simulink model "controller_lab4"  (R2024a)
settings: Solver=FixedStepAuto  StartTime=0.0  StopTime=120  FixedStep=1/100  RelTol=1e-3  EnableMultiTasking=on
settings Model: PacingRate=10  ExtModeTrigDuration=2  Creator=DAUIN-Win10  LastModifiedBy=Alizein Khalifeh
settings OptimizationCC: EnhancedBackFolding=on  PassReuseOutputArgsAs=Individual arguments  ZeroExternalMemoryAtStartup=off  ZeroInternalMemoryAtStartup=off  MaxStackSize=64  OptimizeBlockOrder=speed  DifferentSizesBufferReuse=on  OptimizationCustomize=off  EfficientTunableParamExpr=on
settings DebuggingCC: ParameterOverflowMsg=none  ParameterTunabilityLossMsg=error  UnconnectedInputMsg=warning  UnconnectedOutputMsg=warning  UnconnectedLineMsg=warning
settings HardwareCC: ProdBitPerInt=16  ProdBitPerPointer=16  ProdBitPerSizeT=16  ProdBitPerPtrDiffT=16  ProdLargestAtomicFloat=None  ProdWordSize=8  ProdHWDeviceType=Atmel->AVR
settings ModelReferenceCC: EnableRefExpFcnMdlSchedulingChecks=on
settings SFSimCC: MATLABDynamicMemAlloc=off
settings RTWCC: Description=Embedded Coder  SystemTargetFile=ert.tlc  HardwareBoard=Arduino Uno  TemplateMakefile=ert_default_tmf  Toolchain=Arduino AVR  BuildConfiguration=Faster Runs  GPUComputeCapability=3.5  DLArmComputeVersion=19.05
settings CodeAppCC: ForceParamTrailComments=on  IgnoreCustomStorageClasses=off  OperatorAnnotations=on  SimulinkDataObjDesc=on  SFDataObjDesc=on  InsertBlockDesc=on
settings ERTTargetCC: SupportContinuousTime=on  SupportVariableSizeSignals=on  ExtModeTransport=3  ExtModeStaticAlloc=on  ExtModeAutomaticAllocSize=off  ExtModeStaticAllocSize=250  ExtModeMexFile=ext_xcp  ExtModeIntrfLevel=Level2 - Open

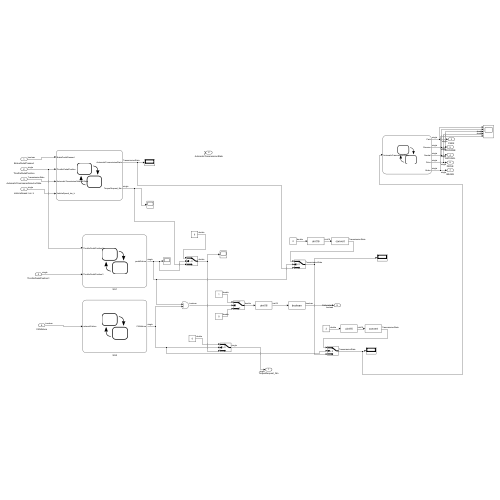
[thumbnail: Simulink's stored preview of the top-level diagram]
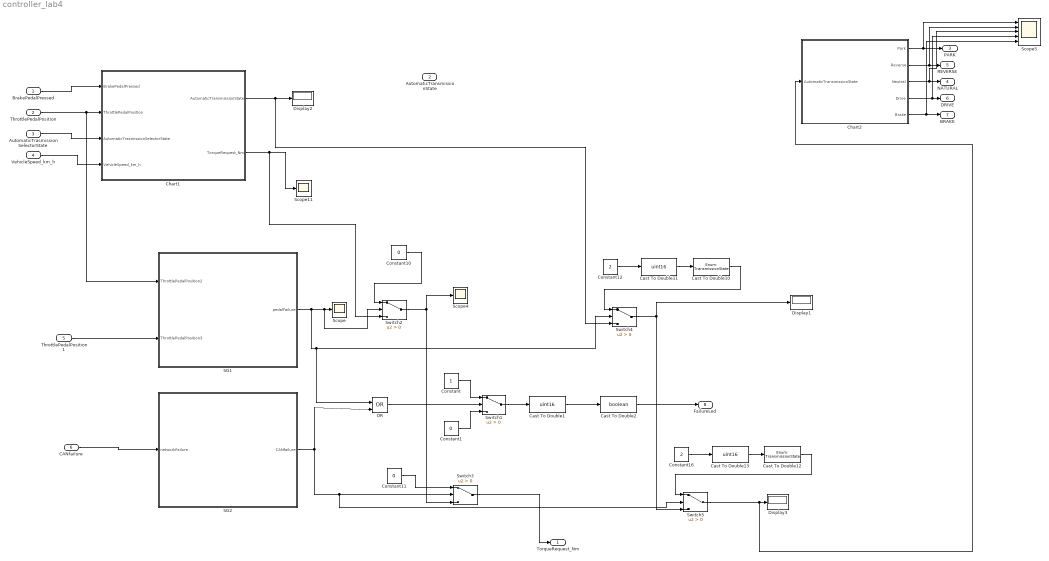
== system controller_lab4 ==
  BrakePedalPressed : Inport  OutDataTypeStr=boolean
  ThrottlePedalPosition : Inport  Port=2  OutDataTypeStr=single
  AutomaticTrasmissionSelectorState : Inport  Port=3  OutDataTypeStr=Enum: TransmissionState
  VehicleSpeed_km_h : Inport  Port=4  OutDataTypeStr=single  Unit=km/h
  ThrottlePedalPosition1 : Inport  Port=5  OutDataTypeStr=single
  CANfailure : Inport  Port=6  OutDataTypeStr=boolean
  Cast To Double1 : DataTypeConversion  OutDataTypeStr=uint16  SaturateOnIntegerOverflow=off  RndMeth=Floor
  Cast To Double10 : DataTypeConversion  OutDataTypeStr=Enum: TransmissionState  SaturateOnIntegerOverflow=off  RndMeth=Floor
  Cast To Double11 : DataTypeConversion  OutDataTypeStr=uint16  SaturateOnIntegerOverflow=off  RndMeth=Floor
  Cast To Double12 : DataTypeConversion  OutDataTypeStr=Enum: TransmissionState  SaturateOnIntegerOverflow=off  RndMeth=Floor
  Cast To Double13 : DataTypeConversion  OutDataTypeStr=uint16  SaturateOnIntegerOverflow=off  RndMeth=Floor
  Cast To Double2 : DataTypeConversion  OutDataTypeStr=boolean  SaturateOnIntegerOverflow=off  RndMeth=Floor
  Chart1 : Stateflow chart  TreatAsAtomicUnit=on
  Chart2 : Stateflow chart  TreatAsAtomicUnit=on
  Constant : Constant
  Constant1 : Constant  Value=0
  Constant10 : Constant  Value=0
  Constant11 : Constant  Value=0
  Constant12 : Constant  Value=2
  Constant16 : Constant  Value=2
  Display1 : Display
  Display2 : Display
  Display3 : Display
  OR : Logic  Operator=OR  IconShape=distinctive  AllPortsSameDT=off  OutDataTypeStr=boolean
  SG1 : Stateflow chart  TreatAsAtomicUnit=on
  SG2 : Stateflow chart  TreatAsAtomicUnit=on
  Scope : Scope
  Scope11 : Scope
  Scope4 : Scope
  Scope5 : Scope  NumInputPorts=5
  Switch{1..5} (5 alike) : Switch  Criteria=u2 > Threshold  SaturateOnIntegerOverflow=off  InputSameDT=off
  TorqueRequest_Nm : Outport  OutDataTypeStr=single  Unit=N*m
  AutomaticTransmissionState : Outport  Port=2
  PARK : Outport  Port=3  OutDataTypeStr=single  Unit=N*m
  NATURAL : Outport  Port=4  OutDataTypeStr=single  Unit=N*m
  REVERSE : Outport  Port=5  OutDataTypeStr=single  Unit=N*m
  DRIVE : Outport  Port=6  OutDataTypeStr=single  Unit=N*m
  BRAKE : Outport  Port=7  OutDataTypeStr=single  Unit=N*m
  FailureLed : Outport  Port=8  OutDataTypeStr=boolean  Unit=N*m
  wires:
  SG1/1(pedalFailure) -> Switch4/2, OR/1, Switch2/2, Scope/1
  Chart2/1(Park) -> Scope5/1, PARK/1
  Chart2/4(Drive) -> Scope5/4, DRIVE/1
  Chart2/5(Brake) -> Scope5/5, BRAKE/1
  Chart1/2(TorqueRequest_Nm) -> Switch2/3, Scope11/1
  Constant10/1 -> Switch2/1
  Constant11/1 -> Switch3/1
  Switch3/1 -> TorqueRequest_Nm/1
  Switch2/1 -> Switch3/3, Scope4/1
  SG2/1(CANfailure) -> Switch5/2, Switch3/2, OR/2
  Switch4/1 -> Display1/1, Switch5/3
  Chart1/1(AutomaticTransmissionState) -> Switch4/3, Display2/1
  Cast To Double11/1 -> Cast To Double10/1
  Switch5/1 -> Chart2/1(AutomaticTransmissionState), Display3/1
  Constant12/1 -> Cast To Double11/1
  Cast To Double10/1 -> Switch4/1
  Constant16/1 -> Cast To Double13/1
  Cast To Double12/1 -> Switch5/1
  Cast To Double13/1 -> Cast To Double12/1
  ThrottlePedalPosition/1 -> SG1/1(ThrottlePedalPosition2), Chart1/2(ThrottlePedalPosition)
  BrakePedalPressed/1 -> Chart1/1(BrakePedalPressed)
  AutomaticTrasmissionSelectorState/1 -> Chart1/3(AutomaticTrasmissionSelectorState)
  VehicleSpeed_km_h/1 -> Chart1/4(VehicleSpeed_km_h)
  ThrottlePedalPosition1/1 -> SG1/2(ThrottlePedalPosition3)
  CANfailure/1 -> SG2/1(networkFailure)
  OR/1 -> Switch1/2
  Constant/1 -> Switch1/1
  Constant1/1 -> Switch1/3
  Switch1/1 -> Cast To Double1/1
  Cast To Double1/1 -> Cast To Double2/1
  Cast To Double2/1 -> FailureLed/1
  Chart2/2(Reverse) -> Scope5/2, REVERSE/1
  Chart2/3(Neutral) -> Scope5/3, NATURAL/1

== stateflow chart controller_lab4/SG1 ==
  (default) -> (junction 14)
  (junction 14) -> (junction 15) [order 1] : [(abs(ThrottlePedalPosition2 - ThrottlePedalPosition3) > 0.05) || (error == 1)]
  (junction 14) -> (junction 16) [order 2] : {pedalFailure = 0;}
  (junction 15) -> (junction 17) : {pedalFailure = 1;error = 1;}
  (junction 17) -> (junction 16)
  (junction 16) -> (junction 18)
  data: ThrottlePedalPosition2 input; ThrottlePedalPosition3 input; pedalFailure output single; error local =0

== stateflow chart controller_lab4/SG2 ==
  (default) -> (junction 14)
  (junction 14) -> (junction 15) [order 1] : [networkFailure == 1 || error == 1]
  (junction 14) -> (junction 16) [order 2] : {CANfailure = 0;}
  (junction 15) -> (junction 17) : {CANfailure = 1; error = 1;}
  (junction 17) -> (junction 16)
  (junction 16) -> (junction 18)
  data: networkFailure input; CANfailure output single; error local =0

== stateflow chart controller_lab4/Chart1 ==
  state P
    entry:
    AutomaticTransmissionState = TransmissionState.Park ;
    TorqueRequest_Nm = 0;
  state B
    entry:
    AutomaticTransmissionState = TransmissionState.Brake ;
    state acceleration
      during:
      TorqueRequest_Nm = T*1.5*(ThrottlePedalPosition-(1/3));
    state braking
      during:
      TorqueRequest_Nm = -T*(1-(3*ThrottlePedalPosition));
    state stop
      entry:
      TorqueRequest_Nm =0;
    (default) -> acceleration
    braking -> acceleration [order 1] : [ThrottlePedalPosition > 1/3 ]
    acceleration -> braking : [ThrottlePedalPosition <= 1/3]
    braking -> stop [order 2] : [VehicleSpeed_km_h <=0]
    stop -> braking [order 2] : [VehicleSpeed_km_h > 0 && ThrottlePedalPosition <= 1/3 ]
    stop -> acceleration [order 1] : [ThrottlePedalPosition > 1/3 ]
  state D
    entry:
    AutomaticTransmissionState = TransmissionState.Drive;
    during:
    TorqueRequest_Nm = T*ThrottlePedalPosition;
  state N
    entry:
    AutomaticTransmissionState = TransmissionState.Neutral;
    TorqueRequest_Nm = 0;
  state R
    entry:
    AutomaticTransmissionState = TransmissionState.Reverse ;
    during:
    TorqueRequest_Nm = -Tr * ThrottlePedalPosition;
  (default) -> P
  N -> P [order 3] : [(abs(VehicleSpeed_km_h) < 5 ) && (BrakePedalPressed ==1) && (AutomaticTrasmissionSelectorState == TransmissionState.Park)]
  P -> N : [(BrakePedalPressed==1) && (AutomaticTrasmissionSelectorState ~= TransmissionState.Park)]
  D -> N [order 2] : [AutomaticTrasmissionSelectorState < TransmissionState.Drive]
  N -> R [order 2] : [(VehicleSpeed_km_h < 5) && (BrakePedalPressed ==1) && (AutomaticTrasmissionSelectorState == TransmissionState.Reverse)]
  B -> D : [(AutomaticTrasmissionSelectorState ~= TransmissionState.Brake) && (ThrottlePedalPosition > 0) ]
  R -> N : [AutomaticTrasmissionSelectorState ~= TransmissionState.Reverse]
  N -> D [order 1] : [(VehicleSpeed_km_h > -5) && (BrakePedalPressed ==1) && (AutomaticTrasmissionSelectorState > TransmissionState.Neutral)]
  D -> B [order 1] : [(ThrottlePedalPosition > (1/3)) && (AutomaticTrasmissionSelectorState == TransmissionState.Brake)]
  data: BrakePedalPressed input boolean; ThrottlePedalPosition input single; AutomaticTrasmissionSelectorState input Enum: TransmissionState; VehicleSpeed_km_h input single; AutomaticTransmissionState output Enum: TransmissionState; TorqueRequest_Nm output single; T local =80; Tr local =40

== stateflow chart controller_lab4/Chart2 ==
  state park
    entry:
    Park = 1;
    Reverse = 0;
    Neutral = 0;
    Drive = 0;
    Brake = 0;
  state neutral
    entry:
    Park = 0;
    Reverse = 0;
    Neutral = 1;
    Drive = 0;
    Brake = 0;
  state brake
    entry:
    Park = 0;
    Reverse = 0;
    Neutral = 0;
    Drive = 0;
    Brake = 1;
  state drive
    entry:
    Park = 0;
    Reverse = 0;
    Neutral = 0;
    Drive = 1;
    Brake = 0;
  state reverse
    entry:
    Park = 0;
    Reverse = 1;
    Neutral = 0;
    Drive = 0;
    Brake = 0;
  (default) -> park
  neutral -> park [order 3] : [AutomaticTransmissionState == TransmissionState.Park ]
  park -> neutral : [AutomaticTransmissionState ~= TransmissionState.Park ]
  drive -> brake [order 1] : [AutomaticTransmissionState == TransmissionState.Brake ]
  neutral -> reverse [order 1] : [AutomaticTransmissionState == TransmissionState.Reverse]
  neutral -> drive [order 2] : [AutomaticTransmissionState > TransmissionState.Neutral ]
  drive -> neutral [order 2] : [AutomaticTransmissionState < TransmissionState.Drive ]
  reverse -> neutral : [AutomaticTransmissionState ~= TransmissionState.Reverse ]
  brake -> drive : [AutomaticTransmissionState ~= TransmissionState.Brake ]
  data: AutomaticTransmissionState input Enum: TransmissionState; Park output single; Reverse output single; Neutral output single; Drive output single; Brake output single
